simulink model "example1"  (R2017a)
settings: Solver=FixedStepAuto  StartTime=0.0  StopTime=10.0  RelTol=1e-3
settings Model: Creator=rober  LastModifiedBy=rober
settings SolverCC: AutoInsertRateTranBlk=on

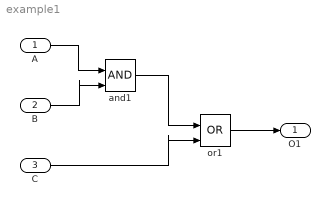
== system example1 ==
  A : Inport  OutDataTypeStr=boolean
  B : Inport  Port=2  OutDataTypeStr=boolean
  C : Inport  Port=3  OutDataTypeStr=boolean
  and1 : Logic  IconShape=distinctive  AllPortsSameDT=off  OutDataTypeStr=boolean
  or1 : Logic  Operator=OR  IconShape=distinctive  AllPortsSameDT=off  OutDataTypeStr=boolean
  O1 : Outport
  wires:
  A/1 -> and1/1
  B/1 -> and1/2
  and1/1 -> or1/1
  C/1 -> or1/2
  or1/1 -> O1/1
